simulink model "Suspension"  (R2018a)
settings: Solver=VariableStepAuto  StartTime=0.0  StopTime=3  RelTol=1e-3
undefined symbols (not defined in the file): cs, ks, kt, ms, mus
settings Model: Creator=adham  LastModifiedBy=adham

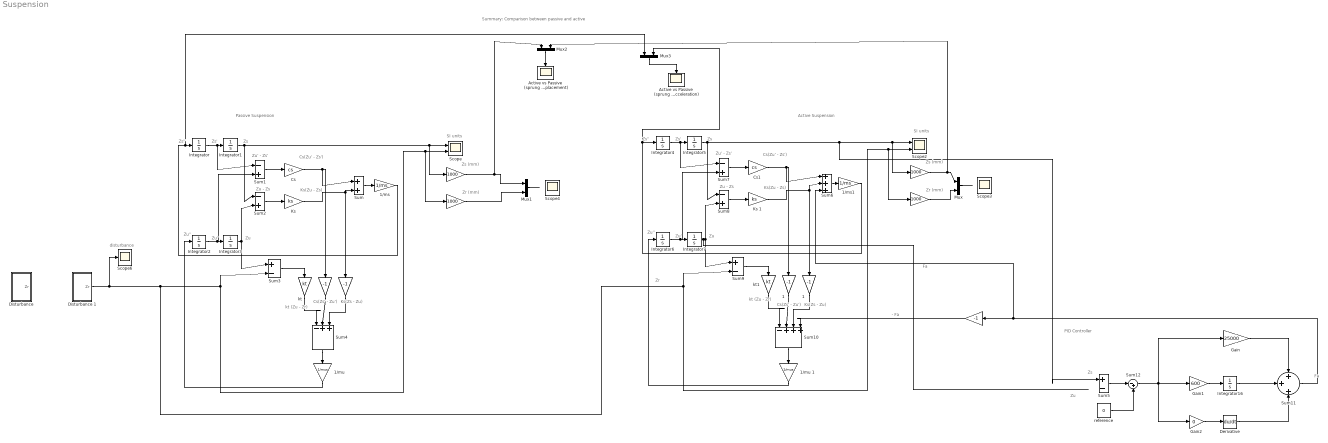
== system Suspension ==
  note: disturbance
  note: Summary: Comparison between passive and active
  note: PID Controller
  note: SI units
  note: Zr
  note: Fa
  note: - Fa
  note: Passive Suspension
  note: kt (Zu - Zr)
  note: Zu' - Zs'
  note: Zs''
  note: Zs'
  note: Zs
  note: Zu''
  note: Zu'
  note: Zu
  note: Cs(Zu' - Zs')
  note: Zu - Zs
  note: Ks(Zu - Zs)
  note: Cs(Zs' - Zu')
  note: Ks(Zs - Zu)
  note: Zs (mm)
  note: Zr (mm)
  note: Zr (mm)
  note: kt (Zu - Zr)
  note: Zu'
  note: Zu''
  note: Zu - Zs
  note: Cs(Zu' - Zs')
  note: Zu' - Zs'
  note: Cs(Zs' - Zu')
  note: Zs''
  note: Ks(Zs - Zu)
  note: Zs'
  note: Zu
  note: Zs
  note: Zs (mm)
  note: Ks(Zu - Zs)
  note: Active Suspension
  note: SI units
  note: Zs
  note: Fa
  note: Zu
   {,,,} (4 alike) : Gain  Gain=1000
   {,,,1,1} (5 alike) : Gain  Gain=-1
  1/ms : Gain  Gain=1/ms
  1/ms1 : Gain  Gain=1/ms
  "1/mu " : Gain  Gain=1/mus
  1/mu 1 : Gain  Gain=1/mus
  Active vs Passive (sprung mass acceleration) : Scope
  Active vs Passive (sprung mass displacement) : Scope
  Cs : Gain  Gain=cs
  Cs1 : Gain  Gain=cs
  Derivative : Derivative
  "Disturbance " : Subsystem
  Disturbance 1 : Subsystem
  Gain : Gain  Gain=25000
  Gain1 : Gain  Gain=600
  Gain2 : Gain  Gain=0
  Integrator{,1..7,16} (9 alike) : Integrator
  "Ks " : Gain  Gain=ks
  Ks 1 : Gain  Gain=ks
  Mux{,1..3} (4 alike) : Mux  Inputs=2
  Scope : Scope  NumInputPorts=2
  Scope2 : Scope  NumInputPorts=2
  Scope3 : Scope
  Scope4 : Scope
  Scope6 : Scope
  Sum : Sum  Inputs=|++
  Sum{1..2,7..8,12} (5 alike) : Sum  Inputs=|-+
  Sum10 : Sum  Inputs=|-+++
  Sum11 : Sum  Inputs=+++
  Sum3 : Sum  Inputs=|+-
  Sum4 : Sum  Inputs=|-++
  Sum5 : Sum  Inputs=|+-
  Sum6 : Sum  Inputs=|+++
  Sum9 : Sum  Inputs=|+-
  kt : Gain  Gain=kt
  kt1 : Gain  Gain=kt
  reference : Constant  Value=0
  wires:
  Integrator/1 -> Sum1/1, Integrator1/1
  Integrator2/1 -> Sum1/2, Integrator3/1
  1/ms/1 -> Mux3/1, Integrator/1
  Sum1/1 -> Cs/1
  Integrator1/1 -> Sum2/1, " "/1, Scope/1
  Sum2/1 -> "Ks "/1
  Cs/1 -> " "/1, Sum/1
  Sum/1 -> 1/ms/1
  "Ks "/1 -> " "/1, Sum/2
  " "/1 -> Sum4/2
  " "/1 -> Sum4/3
  "1/mu "/1 -> Integrator2/1
  Sum3/1 -> kt/1
  kt/1 -> Sum4/1
  Sum4/1 -> "1/mu "/1
  " "/1 -> Mux2/1, Mux1/1
  " "/1 -> Mux1/2
  " "/1 -> Mux2/2, Mux/1
  " "/1 -> Mux/2
  Integrator6/1 -> Sum7/2, Integrator7/1
  Disturbance 1/1(Zr) -> Scope6/1, " "/1, Scope2/2, Sum9/2, " "/1, Scope/2, Sum3/2
  Sum7/1 -> Cs1/1
  kt1/1 -> Sum10/1
  Integrator4/1 -> Sum7/1, Integrator5/1
  1/mu 1/1 -> Integrator6/1
  Cs1/1 -> " 1"/1, Sum6/1
  Ks 1/1 -> " 1"/1, Sum6/2
  " 1"/1 -> Sum10/2
  Sum6/1 -> 1/ms1/1
  Sum8/1 -> Ks 1/1
  Sum10/1 -> 1/mu 1/1
  " 1"/1 -> Sum10/3
  Sum9/1 -> kt1/1
  1/ms1/1 -> Mux3/2, Integrator4/1
  " "/1 -> Sum10/4
  Mux/1 -> ?
  Mux1/1 -> ?
  Sum11/1 -> Sum6/3, " "/1
  reference/1 -> Sum12/2
  Gain1/1 -> Integrator16/1
  Integrator16/1 -> Sum11/2
  Derivative/1 -> Sum11/3
  Gain2/1 -> Derivative/1
  Sum12/1 -> Gain2/1, Gain/1, Gain1/1
  Gain/1 -> Sum11/1
  Integrator5/1 -> Sum8/1, Sum5/1, " "/1, Scope2/1
  Sum5/1 -> Sum12/1
  Mux2/1 -> Active vs Passive (sprung mass displacement)/1
  Integrator3/1 -> Sum3/1, Sum2/2
  Integrator7/1 -> Sum9/1, Sum8/2
  Mux3/1 -> Active vs Passive (sprung mass acceleration)/1

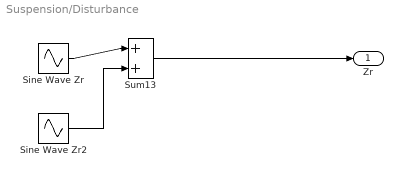
== system Suspension/Disturbance  ==
  Sine Wave Zr : Sin  Amplitude=0.1  Frequency=4  SampleTime=0
  Sine Wave Zr2 : Sin  Amplitude=0.2  Frequency=0.8  SampleTime=0
  Sum13 : Sum  Inputs=|++
  Zr : Outport
  wires:
  Sum13/1 -> Zr/1
  Sine Wave Zr/1 -> Sum13/1
  Sine Wave Zr2/1 -> Sum13/2

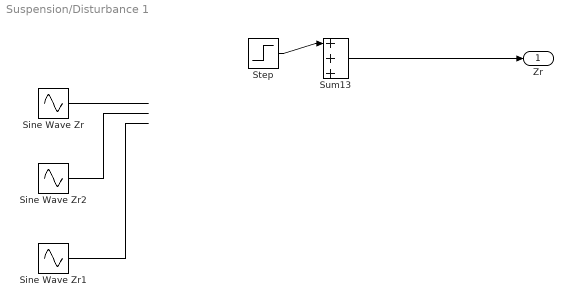
== system Suspension/Disturbance 1 ==
  Sine Wave Zr : Sin  Amplitude=0.2  Frequency=6  SampleTime=0
  Sine Wave Zr1 : Sin  Amplitude=0.01  Frequency=8  SampleTime=0
  Sine Wave Zr2 : Sin  Amplitude=0.2  Frequency=0.8  SampleTime=0
  Step : Step  After=0.1  SampleTime=0
  Sum13 : Sum  Inputs=|+++
  Zr : Outport
  wires:
  Sum13/1 -> Zr/1
  Sine Wave Zr1/1 -> ?
  Sine Wave Zr/1 -> ?
  Sine Wave Zr2/1 -> ?
  Step/1 -> Sum13/1
